simulink model "verify_layerwall_dynamic_mdl"  (R2016b)
settings: Solver=ode45  StartTime=-365*24*3600  StopTime=365*24*3600  MaxStep=3600  RelTol=1e-5  EnableMultiTasking=on
libraries: carnot x1
settings Model: Creator=drhf  LastModifiedBy=drhf
settings DataIOCC: SaveFormat=Array
settings OptimizationCC: DefaultParameterBehavior=Inlined  LifeSpan=inf
settings DebuggingCC: UnderspecifiedInitializationDetection=Classic  MergeDetectMultiDrivingBlocksExec=none  SolverPrmCheckMsg=warning  SFUnexpectedBacktrackingDiag=warning  SFNoUnconditionalDefaultTransitionDiag=warning  SFExecutionAtInitializationDiag=none
settings HardwareCC: ProdBitPerPointer=32  ProdBitPerSizeT=32  ProdBitPerPtrDiffT=32  ProdLargestAtomicFloat=None  ProdIntDivRoundTo=Undefined  ProdEndianess=Unspecified  ProdWordSize=32  ProdHWDeviceType=32-bit Generic
settings ModelReferenceCC: PropagateSignalLabelsOutOfModel=off
settings GRTTargetCC: TargetLangStandard=C89/C90 (ANSI)  GeneratePreprocessorConditionals=Disable all
settings ConfigComp: CovMetricSettings=dw  CovHtmlReporting=on  CovSaveCumulativeToWorkspaceVar=on  CovSaveSingleToWorkspaceVar=on  CovExternalEMLEnable=off

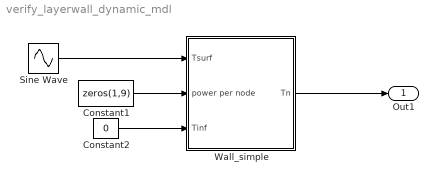
== system verify_layerwall_dynamic_mdl ==
  Constant1 : Constant  Value=zeros(1,9)
  Constant2 : Constant  Value=0
  Sine Wave : Sin  Amplitude=10  Frequency=2*pi/(3600*8760)  Phase=1.5*pi  SampleTime=0
  Wall_simple : Subsystem  mask(simplified wall){wallsize=[1 1], d=ones(1,10)*1, cond=ones(1,10)*1, cwall=ones(1,10)*1000, rho=ones(1,10)*2000, emission_in=1, dactive=1:9, t0=0, tau=100*3600}
      mask prompts: wallsize "size of wall [m] [height width]"; d "thickness of layers [m] (vector) (0 = towards this room)"; cond "conductivity of layers [W/(m*K)] (vector)"; cwall "capacity of layers [J/(kg*K)] (vector)"; rho "density of layers [kg/m³]"; emission_in "emission of wall surface"; dactive "depth active layer in m from inner surface  (-1 = none)"; t0 "initial temperature [degree centigrade]"; tau "time-constant of wall [s]"
      mask help: simplified model to test wall_basic
      mask init:
      | position = [0 90 0 ];
      | % nodes = length(d);
      | wallheight = wallsize(1);
      | wallsurface = wallsize(1)*wallsize(2);
      | 
      | if (dactive>=0) 
      |     active = 1;
      | else
      |     active = 0;
      | end
  Out1 : Outport
  wires:
  Sine Wave/1 -> Wall_simple/1(Tsurf)
  Wall_simple/1(Tn) -> Out1/1
  Constant1/1 -> Wall_simple/2(power per node)
  Constant2/1 -> Wall_simple/3(Tinf)

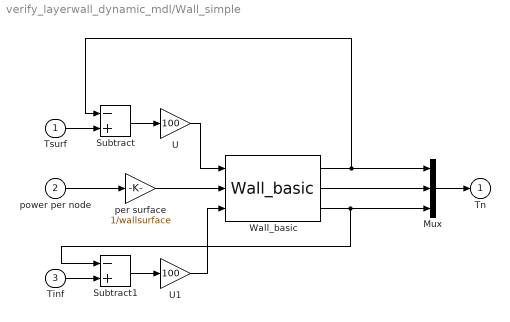
== system verify_layerwall_dynamic_mdl/Wall_simple ==
  Tsurf : Inport
  power per node : Inport  Port=2
  Tinf : Inport  Port=3
  Mux : Mux  Inputs=3
  Subtract : Sum  Inputs=-+
  Subtract1 : Sum  Inputs=-+
  U : Gain  Gain=100  SaturateOnIntegerOverflow=on  OutDataTypeStr=Inherit: Same as input  ParamDataTypeStr=Inherit: Same as input
  U1 : Gain  Gain=100  SaturateOnIntegerOverflow=on  OutDataTypeStr=Inherit: Same as input  ParamDataTypeStr=Inherit: Same as input
  Wall_basic : carnot/Basic/Thermal_Models/Wall_basic  tau=tau  t0=t0  d=d  dactive=dactive  cond=cond  cwall=cwall  rho=rho
  per surface : Gain  Gain=1/wallsurface  SaturateOnIntegerOverflow=on  OutDataTypeStr=Inherit: Same as input  ParamDataTypeStr=Inherit: Same as input
  Tn : Outport
  wires:
  power per node/1 -> per surface/1
  per surface/1 -> Wall_basic/2
  Wall_basic/1 -> Subtract/1, Mux/1
  Wall_basic/3 -> Subtract1/1, Mux/3
  Wall_basic/2 -> Mux/2
  Mux/1 -> Tn/1
  Tsurf/1 -> Subtract/2
  Subtract/1 -> U/1
  U/1 -> Wall_basic/1
  Subtract1/1 -> U1/1
  Tinf/1 -> Subtract1/2
  U1/1 -> Wall_basic/3
